simulink model "quartercar_augmented"  (R2020b)
settings: Solver=ode45  StartTime=0.0  StopTime=5  RelTol=1e-3
values from neighbouring files (symbols this model uses):
  B_f = 1189    [halfcarparameters.mat]
  filter_H = ss(H)    [halfcaraugmented.m]
  K = lqr(A,B,Q_pd,rho_pd)    [accel_jerk_ctrl_testbed.m]    (also in quartersuspensionscript.m)
  K_f = 66793    [halfcarparameters.mat]
  K_tf = 201021    [halfcarparameters.mat]
  m_s = 879.35    [halfcarparameters.mat]
  m_uf = 43.76    [halfcarparameters.mat]
settings Model: Creator=anishabhangui  LastModifiedBy=anishabhangui

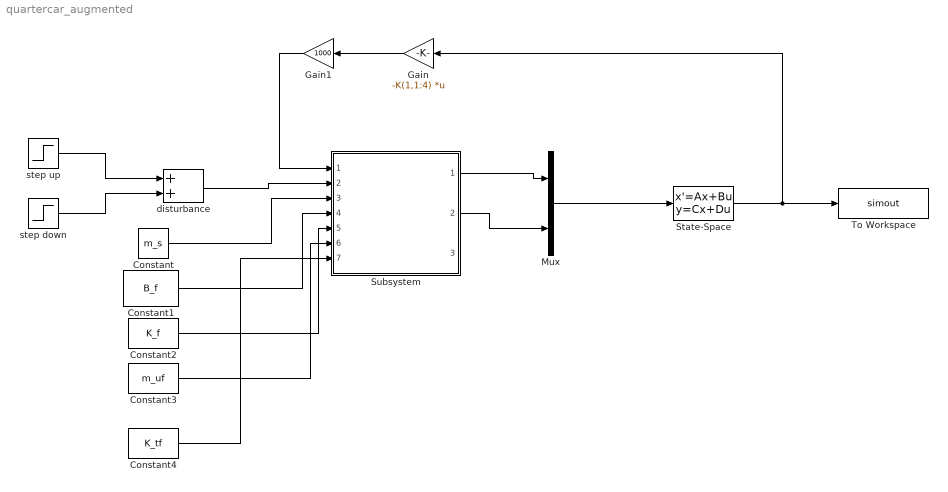
== system quartercar_augmented ==
  Constant : Constant  Value=m_s
  Constant1 : Constant  Value=B_f
  Constant2 : Constant  Value=K_f
  Constant3 : Constant  Value=m_uf
  Constant4 : Constant  Value=K_tf
  Gain : Gain  Gain=-K(1,1:4)  Multiplication=Matrix(K*u)
  Gain1 : Gain  Gain=1000
  Mux : Mux  Inputs=2
  State-Space : StateSpace  A=filter_H.A  B=filter_H.B  C=filter_H.C  D=filter_H.D  InitialCondition=0
  Subsystem : Subsystem  TreatAsAtomicUnit=on  ReferencedSubsystem=quarter_car_w_tire_subsystem
  To Workspace : ToWorkspace  VariableName=simout  SaveFormat=Timeseries  SampleTime=-1
  disturbance : Sum
  step down : Step  After=-1  SampleTime=0
  step up : Step  Time=0  SampleTime=0
  wires:
  Constant/1 -> Subsystem/3
  Constant4/1 -> Subsystem/7
  Constant1/1 -> Subsystem/4
  Constant2/1 -> Subsystem/5
  Constant3/1 -> Subsystem/6
  Subsystem/2 -> Mux/2
  disturbance/1 -> Subsystem/2
  step up/1 -> disturbance/1
  step down/1 -> disturbance/2
  Gain1/1 -> Subsystem/1
  Gain/1 -> Gain1/1
  Subsystem/1 -> Mux/1
  Mux/1 -> State-Space/1
  State-Space/1 -> To Workspace/1, Gain/1
